simulink model "meta_fpb"  (R2015a)
settings: Solver=ode45  StartTime=0.0  StopTime=5  RelTol=1e-3
libraries: dsparch4 x1, simulink x1
settings Model: Creator=User  LastModifiedBy=User

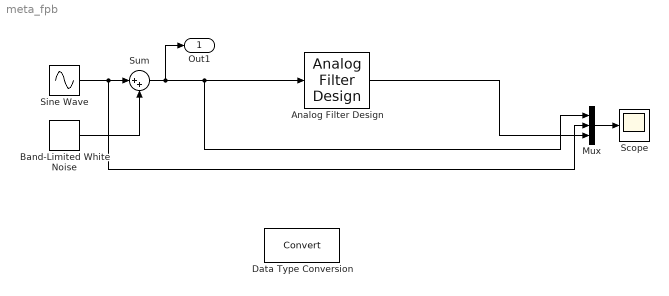
== system meta_fpb ==
  Analog Filter Design : dsparch4/Analog Filter Design  method=Butterworth  filttype=Lowpass  N=3  Wlo=2000*pi  Whi=80  Rp=2  Rs=40
  Band-Limited White Noise : simulink/Sources/Band-Limited White Noise  Cov=[0.0001]  Ts=0.1  seed=[23341]
  Data Type Conversion : DataTypeConversion
  Mux : Mux  Inputs=3
  Scope : Scope
      settings: TimeRange=5
  Sine Wave : Sin  Frequency=2000*pi  SampleTime=0
  Sum : Sum  Inputs=|++
  Out1 : Outport
  wires:
  Mux/1 -> Scope/1
  Analog Filter Design/1 -> Mux/3
  Band-Limited White Noise/1 -> Sum/2
  Sum/1 -> Out1/1, Mux/1, Analog Filter Design/1
  Sine Wave/1 -> Mux/2, Sum/1
